simulink model "l512_devel_pps_2016f"  (R2012b)
settings: Solver=ode45  StartTime=0.0  StopTime=15000  RelTol=1e-3
undefined symbols (not defined in the file): sfp
libraries: xbsIndex_r4 x7383, casper_library_misc x259, casper_library_delays x118, xps_library x12, simulink x1
(part 14 of 82)

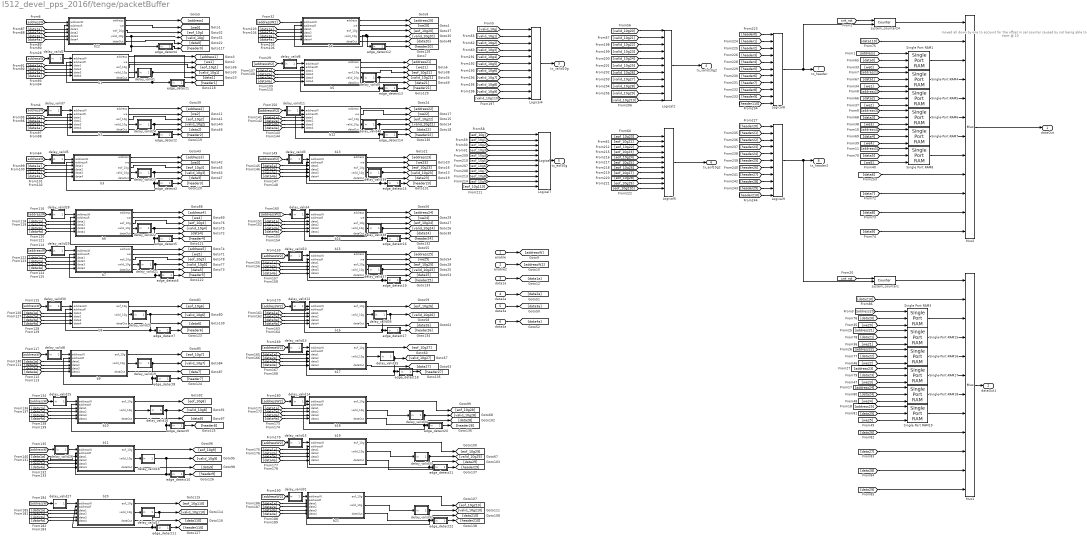
== system l512_devel_pps_2016f/tenge/packetBuffer ==
  note: moved all
      | down by one to account
      | for the offset in sel counter
      | caused by not being able to start @ 10
  enable : Inport
  enable2 : Inport  Port=2
  data1a : Inport  Port=3
  data2a : Inport  Port=4
  data3a : Inport  Port=5
  data4a : Inport  Port=6
  Logical{2,4,6..7} (4 alike) : xbsIndex_r4/Logical  logical_function=OR  inputs=11  en=off  latency=10  precision=Full  arith_type=Unsigned  n_bits=16  bin_pt=0  align_bp=on  dbl_ovrd=off  block_type=logical
      settings: block_version=11.4
  Logical8 : xbsIndex_r4/Logical  logical_function=OR  inputs=11  en=off  latency=5  precision=Full  arith_type=Unsigned  n_bits=16  bin_pt=0  align_bp=on  dbl_ovrd=off  block_type=logical
      settings: block_version=11.4
  Logical9 : xbsIndex_r4/Logical  logical_function=OR  inputs=11  en=off  latency=5  precision=Full  arith_type=Unsigned  n_bits=16  bin_pt=0  align_bp=on  dbl_ovrd=off  block_type=logical
      settings: block_version=11.4
  Mux1 : xbsIndex_r4/Mux  inputs=11  en=off  latency=2  precision=Full  arith_type="Signed  (2's comp)"  n_bits=8  bin_pt=2  quantization=Truncate  overflow=Wrap  dbl_ovrd=off  block_type=mux
      settings: xl_area=[0, 0, 0, 0, 0, 0, 0]
  Mux2 : xbsIndex_r4/Mux  inputs=11  en=off  latency=2  precision=Full  arith_type="Signed  (2's comp)"  n_bits=8  bin_pt=2  quantization=Truncate  overflow=Wrap  dbl_ovrd=off  block_type=mux
      settings: xl_area=[0, 0, 0, 0, 0, 0, 0]
  Single Port RAM{1,3..8,15..19} (12 alike) : xbsIndex_r4/Single Port RAM  depth=872  initVector=0  distributed_mem=Block RAM  write_mode=No Read On Write  rst=off  init_reg=0  en=off  latency=4  dbl_ovrd=off  optimize=Area  block_type=spram
  b1 : Subsystem
  b10 : Subsystem
  b11 : Subsystem
  b12 : Subsystem
  b13 : Subsystem
  b14 : Subsystem
  b15 : Subsystem
  b16 : Subsystem
  b17 : Subsystem
  b18 : Subsystem
  b19 : Subsystem
  b2 : Subsystem
  b20 : Subsystem
  b21 : Subsystem
  b22 : Subsystem
  b3 : Subsystem
  b4 : Subsystem
  b5 : Subsystem
  b6 : Subsystem
  b7 : Subsystem
  b8 : Subsystem
  b9 : Subsystem
  delay_valid1 : Subsystem  mask{delay=1166}
      mask prompts: delay "desired delay (>2)"
      mask Display: fprintf('Z^-%d', delay)
  delay_valid10 : Subsystem  mask{delay=1090}
      mask prompts: delay "desired delay (>2)"
      mask Display: fprintf('Z^-%d', delay)
  delay_valid11 : Subsystem  mask{delay=436}
      mask prompts: delay "desired delay (>2)"
      mask Display: fprintf('Z^-%d', delay)
  delay_valid12 : Subsystem  mask{delay=1308}
      mask prompts: delay "desired delay (>2)"
      mask Display: fprintf('Z^-%d', delay)
  delay_valid13 : Subsystem  mask{delay=1526}
      mask prompts: delay "desired delay (>2)"
      mask Display: fprintf('Z^-%d', delay)
  delay_valid14 : Subsystem  mask{delay=1744}
      mask prompts: delay "desired delay (>2)"
      mask Display: fprintf('Z^-%d', delay)
  delay_valid15 : Subsystem  mask{delay=1962}
      mask prompts: delay "desired delay (>2)"
      mask Display: fprintf('Z^-%d', delay)
  delay_valid16 : Subsystem  mask{delay=9328}
      mask prompts: delay "desired delay (>2)"
      mask Display: fprintf('Z^-%d', delay)
  delay_valid17 : Subsystem  mask{delay=11660}
      mask prompts: delay "desired delay (>2)"
      mask Display: fprintf('Z^-%d', delay)
  delay_valid18 : Subsystem  mask{delay=10494}
      mask prompts: delay "desired delay (>2)"
      mask Display: fprintf('Z^-%d', delay)
  delay_valid19 : Subsystem  mask{delay=8162}
      mask prompts: delay "desired delay (>2)"
      mask Display: fprintf('Z^-%d', delay)
  delay_valid2 : Subsystem  mask{delay=218}
      mask prompts: delay "desired delay (>2)"
      mask Display: fprintf('Z^-%d', delay)
  delay_valid20 : Subsystem  mask{delay=6996}
      mask prompts: delay "desired delay (>2)"
      mask Display: fprintf('Z^-%d', delay)
  delay_valid21 : Subsystem  mask{delay=5830}
      mask prompts: delay "desired delay (>2)"
      mask Display: fprintf('Z^-%d', delay)
  delay_valid22 : Subsystem  mask{delay=4664}
      mask prompts: delay "desired delay (>2)"
      mask Display: fprintf('Z^-%d', delay)
  delay_valid23 : Subsystem  mask{delay=3498}
      mask prompts: delay "desired delay (>2)"
      mask Display: fprintf('Z^-%d', delay)
  delay_valid24 : Subsystem  mask{delay=2332}
      mask prompts: delay "desired delay (>2)"
      mask Display: fprintf('Z^-%d', delay)
  delay_valid25 : Subsystem  mask{delay=1744}
      mask prompts: delay "desired delay (>2)"
      mask Display: fprintf('Z^-%d', delay)
  delay_valid26 : Subsystem  mask{delay=1962}
      mask prompts: delay "desired delay (>2)"
      mask Display: fprintf('Z^-%d', delay)
  delay_valid27 : Subsystem  mask{delay=2180}
      mask prompts: delay "desired delay (>2)"
      mask Display: fprintf('Z^-%d', delay)
  delay_valid28 : Subsystem  mask{delay=872}
      mask prompts: delay "desired delay (>2)"
      mask Display: fprintf('Z^-%d', delay)
  delay_valid29 : Subsystem  mask{delay=1090}
      mask prompts: delay "desired delay (>2)"
      mask Display: fprintf('Z^-%d', delay)
  delay_valid3 : Subsystem  mask{delay=654}
      mask prompts: delay "desired delay (>2)"
      mask Display: fprintf('Z^-%d', delay)
  delay_valid30 : Subsystem  mask{delay=1308}
      mask prompts: delay "desired delay (>2)"
      mask Display: fprintf('Z^-%d', delay)
  delay_valid31 : Subsystem  mask{delay=2180}
      mask prompts: delay "desired delay (>2)"
      mask Display: fprintf('Z^-%d', delay)
  delay_valid32 : Subsystem  mask{delay=11660}
      mask prompts: delay "desired delay (>2)"
      mask Display: fprintf('Z^-%d', delay)
  delay_valid33 : Subsystem  mask{delay=10494}
      mask prompts: delay "desired delay (>2)"
      mask Display: fprintf('Z^-%d', delay)
  delay_valid34 : Subsystem  mask{delay=9328}
      mask prompts: delay "desired delay (>2)"
      mask Display: fprintf('Z^-%d', delay)
  delay_valid35 : Subsystem  mask{delay=8162}
      mask prompts: delay "desired delay (>2)"
      mask Display: fprintf('Z^-%d', delay)
  delay_valid36 : Subsystem  mask{delay=6996}
      mask prompts: delay "desired delay (>2)"
      mask Display: fprintf('Z^-%d', delay)
  delay_valid37 : Subsystem  mask{delay=5830}
      mask prompts: delay "desired delay (>2)"
      mask Display: fprintf('Z^-%d', delay)
  delay_valid38 : Subsystem  mask{delay=4664}
      mask prompts: delay "desired delay (>2)"
      mask Display: fprintf('Z^-%d', delay)
  delay_valid39 : Subsystem  mask{delay=3498}
      mask prompts: delay "desired delay (>2)"
      mask Display: fprintf('Z^-%d', delay)
  delay_valid4 : Subsystem  mask{delay=872}
      mask prompts: delay "desired delay (>2)"
      mask Display: fprintf('Z^-%d', delay)
  delay_valid40 : Subsystem  mask{delay=2332}
      mask prompts: delay "desired delay (>2)"
      mask Display: fprintf('Z^-%d', delay)
  delay_valid5 : Subsystem  mask{delay=654}
      mask prompts: delay "desired delay (>2)"
      mask Display: fprintf('Z^-%d', delay)
  delay_valid6 : Subsystem  mask{delay=218}
      mask prompts: delay "desired delay (>2)"
      mask Display: fprintf('Z^-%d', delay)
  delay_valid7 : Subsystem  mask{delay=436}
      mask prompts: delay "desired delay (>2)"
      mask Display: fprintf('Z^-%d', delay)
  delay_valid8 : Subsystem  mask{delay=1526}
      mask prompts: delay "desired delay (>2)"
      mask Display: fprintf('Z^-%d', delay)
  delay_valid9 : Subsystem  mask{delay=1166}
      mask prompts: delay "desired delay (>2)"
      mask Display: fprintf('Z^-%d', delay)
  edge_detect1 : Subsystem  AncestorBlock=casper_library_misc/edge_detect  mask(edge_detect){edge=Rising, polarity=Active High, x_in=[0 0.08 0.08 0.16 0.16 0.24 0.24 0.32 0.32 0.4], y_in=[-1 -1  1  1  1  1  1  1  1  1], x_out=[0.6 0.68 0.68 0.76 0.76 0.84 0.84 0.92 0.92 1], y_out=[-1 -1  1  1 -1 -1 -1 -1 -1 -1]}
      mask prompts: edge "Edge Type"; polarity "Output Polarity"; x_in "Input X Positions"; y_in "Input Y Positions"; x_out "Output X Positions"; y_out "Output Y Positions"
      mask help: Output is active for one-cycle after each edge of the specified type (i.e. rising, falling or both).
      mask init: same as l512_devel_pps_2016f/tenge/chSel/edge_detect2
      settings: AttributesFormatString=|
      | rising edges
      | active high
      mask Help: Output is active for one-cycle after each edge of the specified type (i.e. rising, falling, or both).  Latency is zero.
      mask TypeOptions edge: Rising | Falling | Both
      mask TypeOptions polarity: Active High | Active Low
      mask Display:
      | plot(x_in_num,0.5+y_in_num*0.2);
      | plot(x_out_num,0.5+y_out_num*0.2);
  edge_detect10 : Subsystem  AncestorBlock=casper_library_misc/edge_detect  mask(edge_detect){edge=Rising, polarity=Active High, x_in=[0 0.08 0.08 0.16 0.16 0.24 0.24 0.32 0.32 0.4], y_in=[-1 -1  1  1  1  1  1  1  1  1], x_out=[0.6 0.68 0.68 0.76 0.76 0.84 0.84 0.92 0.92 1], y_out=[-1 -1  1  1 -1 -1 -1 -1 -1 -1]}
      mask prompts: edge "Edge Type"; polarity "Output Polarity"; x_in "Input X Positions"; y_in "Input Y Positions"; x_out "Output X Positions"; y_out "Output Y Positions"
      mask help: Output is active for one-cycle after each edge of the specified type (i.e. rising, falling or both).
      mask init: same as l512_devel_pps_2016f/tenge/chSel/edge_detect2
      settings: AttributesFormatString=|
      | rising edges
      | active high
      mask Help: Output is active for one-cycle after each edge of the specified type (i.e. rising, falling, or both).  Latency is zero.
      mask TypeOptions edge: Rising | Falling | Both
      mask TypeOptions polarity: Active High | Active Low
      mask Display:
      | plot(x_in_num,0.5+y_in_num*0.2);
      | plot(x_out_num,0.5+y_out_num*0.2);
  edge_detect11 : Subsystem  AncestorBlock=casper_library_misc/edge_detect  mask(edge_detect){edge=Rising, polarity=Active High, x_in=[0 0.08 0.08 0.16 0.16 0.24 0.24 0.32 0.32 0.4], y_in=[-1 -1  1  1  1  1  1  1  1  1], x_out=[0.6 0.68 0.68 0.76 0.76 0.84 0.84 0.92 0.92 1], y_out=[-1 -1  1  1 -1 -1 -1 -1 -1 -1]}
      mask prompts: edge "Edge Type"; polarity "Output Polarity"; x_in "Input X Positions"; y_in "Input Y Positions"; x_out "Output X Positions"; y_out "Output Y Positions"
      mask help: Output is active for one-cycle after each edge of the specified type (i.e. rising, falling or both).
      mask init: same as l512_devel_pps_2016f/tenge/chSel/edge_detect2
      settings: AttributesFormatString=|
      | rising edges
      | active high
      mask Help: Output is active for one-cycle after each edge of the specified type (i.e. rising, falling, or both).  Latency is zero.
      mask TypeOptions edge: Rising | Falling | Both
      mask TypeOptions polarity: Active High | Active Low
      mask Display:
      | plot(x_in_num,0.5+y_in_num*0.2);
      | plot(x_out_num,0.5+y_out_num*0.2);
  edge_detect12 : Subsystem  AncestorBlock=casper_library_misc/edge_detect  mask(edge_detect){edge=Rising, polarity=Active High, x_in=[0 0.08 0.08 0.16 0.16 0.24 0.24 0.32 0.32 0.4], y_in=[-1 -1  1  1  1  1  1  1  1  1], x_out=[0.6 0.68 0.68 0.76 0.76 0.84 0.84 0.92 0.92 1], y_out=[-1 -1  1  1 -1 -1 -1 -1 -1 -1]}
      mask prompts: edge "Edge Type"; polarity "Output Polarity"; x_in "Input X Positions"; y_in "Input Y Positions"; x_out "Output X Positions"; y_out "Output Y Positions"
      mask help: Output is active for one-cycle after each edge of the specified type (i.e. rising, falling or both).
      mask init: same as l512_devel_pps_2016f/tenge/chSel/edge_detect2
      settings: AttributesFormatString=|
      | rising edges
      | active high
      mask Help: Output is active for one-cycle after each edge of the specified type (i.e. rising, falling, or both).  Latency is zero.
      mask TypeOptions edge: Rising | Falling | Both
      mask TypeOptions polarity: Active High | Active Low
      mask Display:
      | plot(x_in_num,0.5+y_in_num*0.2);
      | plot(x_out_num,0.5+y_out_num*0.2);
  edge_detect13 : Subsystem  AncestorBlock=casper_library_misc/edge_detect  mask(edge_detect){edge=Rising, polarity=Active High, x_in=[0 0.08 0.08 0.16 0.16 0.24 0.24 0.32 0.32 0.4], y_in=[-1 -1  1  1  1  1  1  1  1  1], x_out=[0.6 0.68 0.68 0.76 0.76 0.84 0.84 0.92 0.92 1], y_out=[-1 -1  1  1 -1 -1 -1 -1 -1 -1]}
      mask prompts: edge "Edge Type"; polarity "Output Polarity"; x_in "Input X Positions"; y_in "Input Y Positions"; x_out "Output X Positions"; y_out "Output Y Positions"
      mask help: Output is active for one-cycle after each edge of the specified type (i.e. rising, falling or both).
      mask init: same as l512_devel_pps_2016f/tenge/chSel/edge_detect2
      settings: AttributesFormatString=|
      | rising edges
      | active high
      mask Help: Output is active for one-cycle after each edge of the specified type (i.e. rising, falling, or both).  Latency is zero.
      mask TypeOptions edge: Rising | Falling | Both
      mask TypeOptions polarity: Active High | Active Low
      mask Display:
      | plot(x_in_num,0.5+y_in_num*0.2);
      | plot(x_out_num,0.5+y_out_num*0.2);
  edge_detect14 : Subsystem  AncestorBlock=casper_library_misc/edge_detect  mask(edge_detect){edge=Rising, polarity=Active High, x_in=[0 0.08 0.08 0.16 0.16 0.24 0.24 0.32 0.32 0.4], y_in=[-1 -1  1  1  1  1  1  1  1  1], x_out=[0.6 0.68 0.68 0.76 0.76 0.84 0.84 0.92 0.92 1], y_out=[-1 -1  1  1 -1 -1 -1 -1 -1 -1]}
      mask prompts: edge "Edge Type"; polarity "Output Polarity"; x_in "Input X Positions"; y_in "Input Y Positions"; x_out "Output X Positions"; y_out "Output Y Positions"
      mask help: Output is active for one-cycle after each edge of the specified type (i.e. rising, falling or both).
      mask init: same as l512_devel_pps_2016f/tenge/chSel/edge_detect2
      settings: AttributesFormatString=|
      | rising edges
      | active high
      mask Help: Output is active for one-cycle after each edge of the specified type (i.e. rising, falling, or both).  Latency is zero.
      mask TypeOptions edge: Rising | Falling | Both
      mask TypeOptions polarity: Active High | Active Low
      mask Display:
      | plot(x_in_num,0.5+y_in_num*0.2);
      | plot(x_out_num,0.5+y_out_num*0.2);
  edge_detect15 : Subsystem  AncestorBlock=casper_library_misc/edge_detect  mask(edge_detect){edge=Rising, polarity=Active High, x_in=[0 0.08 0.08 0.16 0.16 0.24 0.24 0.32 0.32 0.4], y_in=[-1 -1  1  1  1  1  1  1  1  1], x_out=[0.6 0.68 0.68 0.76 0.76 0.84 0.84 0.92 0.92 1], y_out=[-1 -1  1  1 -1 -1 -1 -1 -1 -1]}
      mask prompts: edge "Edge Type"; polarity "Output Polarity"; x_in "Input X Positions"; y_in "Input Y Positions"; x_out "Output X Positions"; y_out "Output Y Positions"
      mask help: Output is active for one-cycle after each edge of the specified type (i.e. rising, falling or both).
      mask init: same as l512_devel_pps_2016f/tenge/chSel/edge_detect2
      settings: AttributesFormatString=|
      | rising edges
      | active high
      mask Help: Output is active for one-cycle after each edge of the specified type (i.e. rising, falling, or both).  Latency is zero.
      mask TypeOptions edge: Rising | Falling | Both
      mask TypeOptions polarity: Active High | Active Low
      mask Display:
      | plot(x_in_num,0.5+y_in_num*0.2);
      | plot(x_out_num,0.5+y_out_num*0.2);
  edge_detect16 : Subsystem  AncestorBlock=casper_library_misc/edge_detect  mask(edge_detect){edge=Rising, polarity=Active High, x_in=[0 0.08 0.08 0.16 0.16 0.24 0.24 0.32 0.32 0.4], y_in=[-1 -1  1  1  1  1  1  1  1  1], x_out=[0.6 0.68 0.68 0.76 0.76 0.84 0.84 0.92 0.92 1], y_out=[-1 -1  1  1 -1 -1 -1 -1 -1 -1]}
      mask prompts: edge "Edge Type"; polarity "Output Polarity"; x_in "Input X Positions"; y_in "Input Y Positions"; x_out "Output X Positions"; y_out "Output Y Positions"
      mask help: Output is active for one-cycle after each edge of the specified type (i.e. rising, falling or both).
      mask init: same as l512_devel_pps_2016f/tenge/chSel/edge_detect2
      settings: AttributesFormatString=|
      | rising edges
      | active high
      mask Help: Output is active for one-cycle after each edge of the specified type (i.e. rising, falling, or both).  Latency is zero.
      mask TypeOptions edge: Rising | Falling | Both
      mask TypeOptions polarity: Active High | Active Low
      mask Display:
      | plot(x_in_num,0.5+y_in_num*0.2);
      | plot(x_out_num,0.5+y_out_num*0.2);
  edge_detect17 : Subsystem  AncestorBlock=casper_library_misc/edge_detect  mask(edge_detect){edge=Rising, polarity=Active High, x_in=[0 0.08 0.08 0.16 0.16 0.24 0.24 0.32 0.32 0.4], y_in=[-1 -1  1  1  1  1  1  1  1  1], x_out=[0.6 0.68 0.68 0.76 0.76 0.84 0.84 0.92 0.92 1], y_out=[-1 -1  1  1 -1 -1 -1 -1 -1 -1]}
      mask prompts: edge "Edge Type"; polarity "Output Polarity"; x_in "Input X Positions"; y_in "Input Y Positions"; x_out "Output X Positions"; y_out "Output Y Positions"
      mask help: Output is active for one-cycle after each edge of the specified type (i.e. rising, falling or both).
      mask init: same as l512_devel_pps_2016f/tenge/chSel/edge_detect2
      settings: AttributesFormatString=|
      | rising edges
      | active high
      mask Help: Output is active for one-cycle after each edge of the specified type (i.e. rising, falling, or both).  Latency is zero.
      mask TypeOptions edge: Rising | Falling | Both
      mask TypeOptions polarity: Active High | Active Low
      mask Display:
      | plot(x_in_num,0.5+y_in_num*0.2);
      | plot(x_out_num,0.5+y_out_num*0.2);
  edge_detect18 : Subsystem  AncestorBlock=casper_library_misc/edge_detect  mask(edge_detect){edge=Rising, polarity=Active High, x_in=[0 0.08 0.08 0.16 0.16 0.24 0.24 0.32 0.32 0.4], y_in=[-1 -1  1  1  1  1  1  1  1  1], x_out=[0.6 0.68 0.68 0.76 0.76 0.84 0.84 0.92 0.92 1], y_out=[-1 -1  1  1 -1 -1 -1 -1 -1 -1]}
      mask prompts: edge "Edge Type"; polarity "Output Polarity"; x_in "Input X Positions"; y_in "Input Y Positions"; x_out "Output X Positions"; y_out "Output Y Positions"
      mask help: Output is active for one-cycle after each edge of the specified type (i.e. rising, falling or both).
      mask init: same as l512_devel_pps_2016f/tenge/chSel/edge_detect2
      settings: AttributesFormatString=|
      | rising edges
      | active high
      mask Help: Output is active for one-cycle after each edge of the specified type (i.e. rising, falling, or both).  Latency is zero.
      mask TypeOptions edge: Rising | Falling | Both
      mask TypeOptions polarity: Active High | Active Low
      mask Display:
      | plot(x_in_num,0.5+y_in_num*0.2);
      | plot(x_out_num,0.5+y_out_num*0.2);
  edge_detect19 : Subsystem  AncestorBlock=casper_library_misc/edge_detect  mask(edge_detect){edge=Rising, polarity=Active High, x_in=[0 0.08 0.08 0.16 0.16 0.24 0.24 0.32 0.32 0.4], y_in=[-1 -1  1  1  1  1  1  1  1  1], x_out=[0.6 0.68 0.68 0.76 0.76 0.84 0.84 0.92 0.92 1], y_out=[-1 -1  1  1 -1 -1 -1 -1 -1 -1]}
      mask prompts: edge "Edge Type"; polarity "Output Polarity"; x_in "Input X Positions"; y_in "Input Y Positions"; x_out "Output X Positions"; y_out "Output Y Positions"
      mask help: Output is active for one-cycle after each edge of the specified type (i.e. rising, falling or both).
      mask init: same as l512_devel_pps_2016f/tenge/chSel/edge_detect2
      settings: AttributesFormatString=|
      | rising edges
      | active high
      mask Help: Output is active for one-cycle after each edge of the specified type (i.e. rising, falling, or both).  Latency is zero.
      mask TypeOptions edge: Rising | Falling | Both
      mask TypeOptions polarity: Active High | Active Low
      mask Display:
      | plot(x_in_num,0.5+y_in_num*0.2);
      | plot(x_out_num,0.5+y_out_num*0.2);
  edge_detect2 : Subsystem  AncestorBlock=casper_library_misc/edge_detect  mask(edge_detect){edge=Rising, polarity=Active High, x_in=[0 0.08 0.08 0.16 0.16 0.24 0.24 0.32 0.32 0.4], y_in=[-1 -1  1  1  1  1  1  1  1  1], x_out=[0.6 0.68 0.68 0.76 0.76 0.84 0.84 0.92 0.92 1], y_out=[-1 -1  1  1 -1 -1 -1 -1 -1 -1]}
      mask prompts: edge "Edge Type"; polarity "Output Polarity"; x_in "Input X Positions"; y_in "Input Y Positions"; x_out "Output X Positions"; y_out "Output Y Positions"
      mask help: Output is active for one-cycle after each edge of the specified type (i.e. rising, falling or both).
      mask init: same as l512_devel_pps_2016f/tenge/chSel/edge_detect2
      settings: AttributesFormatString=|
      | rising edges
      | active high
      mask Help: Output is active for one-cycle after each edge of the specified type (i.e. rising, falling, or both).  Latency is zero.
      mask TypeOptions edge: Rising | Falling | Both
      mask TypeOptions polarity: Active High | Active Low
      mask Display:
      | plot(x_in_num,0.5+y_in_num*0.2);
      | plot(x_out_num,0.5+y_out_num*0.2);
  edge_detect20 : Subsystem  AncestorBlock=casper_library_misc/edge_detect  mask(edge_detect){edge=Rising, polarity=Active High, x_in=[0 0.08 0.08 0.16 0.16 0.24 0.24 0.32 0.32 0.4], y_in=[-1 -1  1  1  1  1  1  1  1  1], x_out=[0.6 0.68 0.68 0.76 0.76 0.84 0.84 0.92 0.92 1], y_out=[-1 -1  1  1 -1 -1 -1 -1 -1 -1]}
      mask prompts: edge "Edge Type"; polarity "Output Polarity"; x_in "Input X Positions"; y_in "Input Y Positions"; x_out "Output X Positions"; y_out "Output Y Positions"
      mask help: Output is active for one-cycle after each edge of the specified type (i.e. rising, falling or both).
      mask init: same as l512_devel_pps_2016f/tenge/chSel/edge_detect2
      settings: AttributesFormatString=|
      | rising edges
      | active high
      mask Help: Output is active for one-cycle after each edge of the specified type (i.e. rising, falling, or both).  Latency is zero.
      mask TypeOptions edge: Rising | Falling | Both
      mask TypeOptions polarity: Active High | Active Low
      mask Display:
      | plot(x_in_num,0.5+y_in_num*0.2);
      | plot(x_out_num,0.5+y_out_num*0.2);
  edge_detect21 : Subsystem  AncestorBlock=casper_library_misc/edge_detect  mask(edge_detect){edge=Rising, polarity=Active High, x_in=[0 0.08 0.08 0.16 0.16 0.24 0.24 0.32 0.32 0.4], y_in=[-1 -1  1  1  1  1  1  1  1  1], x_out=[0.6 0.68 0.68 0.76 0.76 0.84 0.84 0.92 0.92 1], y_out=[-1 -1  1  1 -1 -1 -1 -1 -1 -1]}
      mask prompts: edge "Edge Type"; polarity "Output Polarity"; x_in "Input X Positions"; y_in "Input Y Positions"; x_out "Output X Positions"; y_out "Output Y Positions"
      mask help: Output is active for one-cycle after each edge of the specified type (i.e. rising, falling or both).
      mask init: same as l512_devel_pps_2016f/tenge/chSel/edge_detect2
      settings: AttributesFormatString=|
      | rising edges
      | active high
      mask Help: Output is active for one-cycle after each edge of the specified type (i.e. rising, falling, or both).  Latency is zero.
      mask TypeOptions edge: Rising | Falling | Both
      mask TypeOptions polarity: Active High | Active Low
      mask Display:
      | plot(x_in_num,0.5+y_in_num*0.2);
      | plot(x_out_num,0.5+y_out_num*0.2);
  edge_detect22 : Subsystem  AncestorBlock=casper_library_misc/edge_detect  mask(edge_detect){edge=Rising, polarity=Active High, x_in=[0 0.08 0.08 0.16 0.16 0.24 0.24 0.32 0.32 0.4], y_in=[-1 -1  1  1  1  1  1  1  1  1], x_out=[0.6 0.68 0.68 0.76 0.76 0.84 0.84 0.92 0.92 1], y_out=[-1 -1  1  1 -1 -1 -1 -1 -1 -1]}
      mask prompts: edge "Edge Type"; polarity "Output Polarity"; x_in "Input X Positions"; y_in "Input Y Positions"; x_out "Output X Positions"; y_out "Output Y Positions"
      mask help: Output is active for one-cycle after each edge of the specified type (i.e. rising, falling or both).
      mask init: same as l512_devel_pps_2016f/tenge/chSel/edge_detect2
      settings: AttributesFormatString=|
      | rising edges
      | active high
      mask Help: Output is active for one-cycle after each edge of the specified type (i.e. rising, falling, or both).  Latency is zero.
      mask TypeOptions edge: Rising | Falling | Both
      mask TypeOptions polarity: Active High | Active Low
      mask Display:
      | plot(x_in_num,0.5+y_in_num*0.2);
      | plot(x_out_num,0.5+y_out_num*0.2);
  edge_detect3 : Subsystem  AncestorBlock=casper_library_misc/edge_detect  mask(edge_detect){edge=Rising, polarity=Active High, x_in=[0 0.08 0.08 0.16 0.16 0.24 0.24 0.32 0.32 0.4], y_in=[-1 -1  1  1  1  1  1  1  1  1], x_out=[0.6 0.68 0.68 0.76 0.76 0.84 0.84 0.92 0.92 1], y_out=[-1 -1  1  1 -1 -1 -1 -1 -1 -1]}
      mask prompts: edge "Edge Type"; polarity "Output Polarity"; x_in "Input X Positions"; y_in "Input Y Positions"; x_out "Output X Positions"; y_out "Output Y Positions"
      mask help: Output is active for one-cycle after each edge of the specified type (i.e. rising, falling or both).
      mask init: same as l512_devel_pps_2016f/tenge/chSel/edge_detect2
      settings: AttributesFormatString=|
      | rising edges
      | active high
      mask Help: Output is active for one-cycle after each edge of the specified type (i.e. rising, falling, or both).  Latency is zero.
      mask TypeOptions edge: Rising | Falling | Both
      mask TypeOptions polarity: Active High | Active Low
      mask Display:
      | plot(x_in_num,0.5+y_in_num*0.2);
      | plot(x_out_num,0.5+y_out_num*0.2);
  edge_detect4 : Subsystem  AncestorBlock=casper_library_misc/edge_detect  mask(edge_detect){edge=Rising, polarity=Active High, x_in=[0 0.08 0.08 0.16 0.16 0.24 0.24 0.32 0.32 0.4], y_in=[-1 -1  1  1  1  1  1  1  1  1], x_out=[0.6 0.68 0.68 0.76 0.76 0.84 0.84 0.92 0.92 1], y_out=[-1 -1  1  1 -1 -1 -1 -1 -1 -1]}
      mask prompts: edge "Edge Type"; polarity "Output Polarity"; x_in "Input X Positions"; y_in "Input Y Positions"; x_out "Output X Positions"; y_out "Output Y Positions"
      mask help: Output is active for one-cycle after each edge of the specified type (i.e. rising, falling or both).
      mask init: same as l512_devel_pps_2016f/tenge/chSel/edge_detect2
      settings: AttributesFormatString=|
      | rising edges
      | active high
      mask Help: Output is active for one-cycle after each edge of the specified type (i.e. rising, falling, or both).  Latency is zero.
      mask TypeOptions edge: Rising | Falling | Both
      mask TypeOptions polarity: Active High | Active Low
      mask Display:
      | plot(x_in_num,0.5+y_in_num*0.2);
      | plot(x_out_num,0.5+y_out_num*0.2);
  edge_detect5 : Subsystem  AncestorBlock=casper_library_misc/edge_detect  mask(edge_detect){edge=Rising, polarity=Active High, x_in=[0 0.08 0.08 0.16 0.16 0.24 0.24 0.32 0.32 0.4], y_in=[-1 -1  1  1  1  1  1  1  1  1], x_out=[0.6 0.68 0.68 0.76 0.76 0.84 0.84 0.92 0.92 1], y_out=[-1 -1  1  1 -1 -1 -1 -1 -1 -1]}
      mask prompts: edge "Edge Type"; polarity "Output Polarity"; x_in "Input X Positions"; y_in "Input Y Positions"; x_out "Output X Positions"; y_out "Output Y Positions"
      mask help: Output is active for one-cycle after each edge of the specified type (i.e. rising, falling or both).
      mask init: same as l512_devel_pps_2016f/tenge/chSel/edge_detect2
      settings: AttributesFormatString=|
      | rising edges
      | active high
      mask Help: Output is active for one-cycle after each edge of the specified type (i.e. rising, falling, or both).  Latency is zero.
      mask TypeOptions edge: Rising | Falling | Both
      mask TypeOptions polarity: Active High | Active Low
      mask Display:
      | plot(x_in_num,0.5+y_in_num*0.2);
      | plot(x_out_num,0.5+y_out_num*0.2);
  edge_detect6 : Subsystem  AncestorBlock=casper_library_misc/edge_detect  mask(edge_detect){edge=Rising, polarity=Active High, x_in=[0 0.08 0.08 0.16 0.16 0.24 0.24 0.32 0.32 0.4], y_in=[-1 -1  1  1  1  1  1  1  1  1], x_out=[0.6 0.68 0.68 0.76 0.76 0.84 0.84 0.92 0.92 1], y_out=[-1 -1  1  1 -1 -1 -1 -1 -1 -1]}
      mask prompts: edge "Edge Type"; polarity "Output Polarity"; x_in "Input X Positions"; y_in "Input Y Positions"; x_out "Output X Positions"; y_out "Output Y Positions"
      mask help: Output is active for one-cycle after each edge of the specified type (i.e. rising, falling or both).
      mask init: same as l512_devel_pps_2016f/tenge/chSel/edge_detect2
      settings: AttributesFormatString=|
      | rising edges
      | active high
      mask Help: Output is active for one-cycle after each edge of the specified type (i.e. rising, falling, or both).  Latency is zero.
      mask TypeOptions edge: Rising | Falling | Both
      mask TypeOptions polarity: Active High | Active Low
      mask Display:
      | plot(x_in_num,0.5+y_in_num*0.2);
      | plot(x_out_num,0.5+y_out_num*0.2);
  edge_detect7 : Subsystem  AncestorBlock=casper_library_misc/edge_detect  mask(edge_detect){edge=Rising, polarity=Active High, x_in=[0 0.08 0.08 0.16 0.16 0.24 0.24 0.32 0.32 0.4], y_in=[-1 -1  1  1  1  1  1  1  1  1], x_out=[0.6 0.68 0.68 0.76 0.76 0.84 0.84 0.92 0.92 1], y_out=[-1 -1  1  1 -1 -1 -1 -1 -1 -1]}
      mask prompts: edge "Edge Type"; polarity "Output Polarity"; x_in "Input X Positions"; y_in "Input Y Positions"; x_out "Output X Positions"; y_out "Output Y Positions"
      mask help: Output is active for one-cycle after each edge of the specified type (i.e. rising, falling or both).
      mask init: same as l512_devel_pps_2016f/tenge/chSel/edge_detect2
      settings: AttributesFormatString=|
      | rising edges
      | active high
      mask Help: Output is active for one-cycle after each edge of the specified type (i.e. rising, falling, or both).  Latency is zero.
      mask TypeOptions edge: Rising | Falling | Both
      mask TypeOptions polarity: Active High | Active Low
      mask Display:
      | plot(x_in_num,0.5+y_in_num*0.2);
      | plot(x_out_num,0.5+y_out_num*0.2);
  edge_detect8 : Subsystem  AncestorBlock=casper_library_misc/edge_detect  mask(edge_detect){edge=Rising, polarity=Active High, x_in=[0 0.08 0.08 0.16 0.16 0.24 0.24 0.32 0.32 0.4], y_in=[-1 -1  1  1  1  1  1  1  1  1], x_out=[0.6 0.68 0.68 0.76 0.76 0.84 0.84 0.92 0.92 1], y_out=[-1 -1  1  1 -1 -1 -1 -1 -1 -1]}
      mask prompts: edge "Edge Type"; polarity "Output Polarity"; x_in "Input X Positions"; y_in "Input Y Positions"; x_out "Output X Positions"; y_out "Output Y Positions"
      mask help: Output is active for one-cycle after each edge of the specified type (i.e. rising, falling or both).
      mask init: same as l512_devel_pps_2016f/tenge/chSel/edge_detect2
      settings: AttributesFormatString=|
      | rising edges
      | active high
      mask Help: Output is active for one-cycle after each edge of the specified type (i.e. rising, falling, or both).  Latency is zero.
      mask TypeOptions edge: Rising | Falling | Both
      mask TypeOptions polarity: Active High | Active Low
      mask Display:
      | plot(x_in_num,0.5+y_in_num*0.2);
      | plot(x_out_num,0.5+y_out_num*0.2);
  edge_detect9 : Subsystem  AncestorBlock=casper_library_misc/edge_detect  mask(edge_detect){edge=Rising, polarity=Active High, x_in=[0 0.08 0.08 0.16 0.16 0.24 0.24 0.32 0.32 0.4], y_in=[-1 -1  1  1  1  1  1  1  1  1], x_out=[0.6 0.68 0.68 0.76 0.76 0.84 0.84 0.92 0.92 1], y_out=[-1 -1  1  1 -1 -1 -1 -1 -1 -1]}
      mask prompts: edge "Edge Type"; polarity "Output Polarity"; x_in "Input X Positions"; y_in "Input Y Positions"; x_out "Output X Positions"; y_out "Output Y Positions"
      mask help: Output is active for one-cycle after each edge of the specified type (i.e. rising, falling or both).
      mask init: same as l512_devel_pps_2016f/tenge/chSel/edge_detect2
      settings: AttributesFormatString=|
      | rising edges
      | active high
      mask Help: Output is active for one-cycle after each edge of the specified type (i.e. rising, falling, or both).  Latency is zero.
      mask TypeOptions edge: Rising | Falling | Both
      mask TypeOptions polarity: Active High | Active Low
      mask Display:
      | plot(x_in_num,0.5+y_in_num*0.2);
      | plot(x_out_num,0.5+y_out_num*0.2);
  system_counter1 : xbsIndex_r4/Counter  cnt_type=Count Limited  cnt_to=10  operation=Up  start_count=0  cnt_by_val=1  arith_type=Unsigned  n_bits=4  bin_pt=0  load_pin=off  rst=on  en=on  explicit_period=on  period=1  dbl_ovrd=off  use_behavioral_HDL=off  implementation=Fabric  block_type=counter
      settings: block_version=11.4
  system_counter24 : xbsIndex_r4/Counter  cnt_type=Count Limited  cnt_to=10  operation=Up  start_count=0  cnt_by_val=1  arith_type=Unsigned  n_bits=4  bin_pt=0  load_pin=off  rst=on  en=on  explicit_period=on  period=1  dbl_ovrd=off  use_behavioral_HDL=off  implementation=Fabric  block_type=counter
      settings: block_version=11.4
  dataOut : Outport
  dataOut1 : Outport  Port=2
  tx_valid10g : Outport  Port=3
  tx_valid10g2 : Outport  Port=4
  tx_eof10g : Outport  Port=5
  tx_eof10g2 : Outport  Port=6
  tx_header : Outport  Port=7
  tx_header2 : Outport  Port=8
  wires:
  [data110] -> Mux2/2
  Single Port RAM1/1 -> Mux2/3
  Single Port RAM4/1 -> Mux2/4
  Single Port RAM5/1 -> Mux2/5
  Single Port RAM6/1 -> Mux2/6
  Single Port RAM7/1 -> Mux2/7
  Single Port RAM8/1 -> Mux2/8
  [data7] -> Mux2/10
  [data8] -> Mux2/11
  [data9] -> Mux2/12
  Mux2/1 -> dataOut/1
  [data210] -> Mux1/2
  Single Port RAM3/1 -> Mux1/3
  Single Port RAM15/1 -> Mux1/4
  Single Port RAM16/1 -> Mux1/5
  Single Port RAM17/1 -> Mux1/6
  Single Port RAM18/1 -> Mux1/7
  Single Port RAM19/1 -> Mux1/8
  [data26] -> Mux1/9
  [data27] -> Mux1/10
  [data28] -> Mux1/11
  [data29] -> Mux1/12
  Mux1/1 -> dataOut1/1
  enable/1 -> [addressW]
  enable2/1 -> [addressW2]
  [addressW] -> b22/1(addressW)
  b22/1(address) -> [address]
  b22/2(we) -> [we0]
  [addressW] -> delay_valid2/1(in)
  b1/1(address) -> [address1]
  b1/2(we) -> [we1]
  b4/1(address) -> [address20]
  [addressW2] -> delay_valid6/1(in)
  [valid_10g] -> Logical4/1
  [valid_10g1] -> Logical4/2
  Logical4/1 -> tx_valid10g/1
  [valid_10g20] -> Logical2/1
  [valid_10g21] -> Logical2/2
  Logical2/1 -> tx_valid10g2/1
  [eof_10g] -> Logical7/1
  [eof_10g1] -> Logical7/2
  Logical7/1 -> tx_eof10g/1
  [eof_10g20] -> Logical6/1
  [eof_10g21] -> Logical6/2
  Logical6/1 -> tx_eof10g2/1
  b4/2(we) -> [we20]
  b1/4(valid_10g) -> delay_valid1/1(in)
  b4/4(valid_10g) -> [valid_10g20], b4/2(addressR), edge_detect12/1(in)
  b4/3(eof_10g) -> [eof_10g20]
  [addressW] -> delay_valid7/1(in)
  b2/1(address) -> [address2]
  b2/2(we) -> [we2]
  b2/4(valid_10g) -> delay_valid24/1(in)
  b2/3(eof_10g) -> [eof_10g2]
  [eof_10g2] -> Logical7/3
  [eof_10g3] -> Logical7/4
  [valid_10g2] -> Logical4/3
  [valid_10g3] -> Logical4/4
  [addressW] -> delay_valid5/1(in)
  delay_valid6/1(out) -> b5/1(addressW)
  delay_valid2/1(out) -> b1/1(addressW)
  [addressW2] -> b4/1(addressW)
  b22/5(dataOut) -> [data0]
  b1/5(dataOut) -> [data1]
  b2/5(dataOut) -> [data2]
  b4/5(dataOut) -> [data20]
  data1a/1 -> [data1a]
  data2a/1 -> [data2a]
  data3a/1 -> [data3a]
  data4a/1 -> [data4a]
  [data1a] -> b22/3(data1)
  [data2a] -> b22/4(data2)
  [data3a] -> b22/5(data3)
  [data4a] -> b22/6(data4)
  [data1a] -> b1/3(data1)
  [data2a] -> b1/4(data2)
  [data3a] -> b1/5(data3)
  [data4a] -> b1/6(data4)
  [data1a] -> b2/3(data1)
  [data2a] -> b2/4(data2)
  [data3a] -> b2/5(data3)
  [data4a] -> b2/6(data4)
  [data1a] -> b3/3(data1)
  [data2a] -> b3/4(data2)
  [data3a] -> b3/5(data3)
  [data4a] -> b3/6(data4)
  [data1a] -> b4/3(data1)
  [data2a] -> b4/4(data2)
  [data3a] -> b4/5(data3)
  [data4a] -> b4/6(data4)
  [data1a] -> b5/3(data1)
  [data2a] -> b5/4(data2)
  [data3a] -> b5/5(data3)
  [data4a] -> b5/6(data4)
  [addressW] -> delay_valid28/1(in)
  [addressW] -> delay_valid29/1(in)
  [addressW] -> delay_valid30/1(in)
  b8/2(valid_10g) -> delay_valid20/1(in)
  b8/1(eof_10g) -> [eof_10g6]
  [addressW] -> delay_valid8/1(in)
  delay_valid29/1(out) -> b7/1(addressW)
  b8/3(dataOut) -> [data6]
  [data1a] -> b6/3(data1)
  [data2a] -> b6/4(data2)
  [data3a] -> b6/5(data3)
  [data4a] -> b6/6(data4)
  [data1a] -> b7/3(data1)
  [data2a] -> b7/4(data2)
  [data3a] -> b7/5(data3)
  [data4a] -> b7/6(data4)
  [data1a] -> b8/3(data1)
  [data2a] -> b8/4(data2)
  [data3a] -> b8/5(data3)
  [data4a] -> b8/6(data4)
  [data1a] -> b9/3(data1)
  [data2a] -> b9/4(data2)
  [data3a] -> b9/5(data3)
  [data4a] -> b9/6(data4)
  [addressW] -> delay_valid25/1(in)
  [addressW] -> delay_valid26/1(in)
  [data1a] -> b10/3(data1)
  [data2a] -> b10/4(data2)
  [data3a] -> b10/5(data3)
  [data4a] -> b10/6(data4)
  [data1a] -> b11/3(data1)
  [data2a] -> b11/4(data2)
  [data3a] -> b11/5(data3)
  [data4a] -> b11/6(data4)
  [addressW2] -> delay_valid3/1(in)
  delay_valid3/1(out) -> b13/1(addressW)
  [addressW2] -> delay_valid11/1(in)
  [data1a] -> b12/3(data1)
  [data2a] -> b12/4(data2)
  [data3a] -> b12/5(data3)
  [data4a] -> b12/6(data4)
  [data1a] -> b13/3(data1)
  [data2a] -> b13/4(data2)
  [data3a] -> b13/5(data3)
  [data4a] -> b13/6(data4)
  [addressW2] -> delay_valid10/1(in)
  delay_valid10/1(out) -> b15/1(addressW)
  [addressW2] -> delay_valid4/1(in)
  [data1a] -> b14/3(data1)
  [data2a] -> b14/4(data2)
  [data3a] -> b14/5(data3)
  [data4a] -> b14/6(data4)
  [data1a] -> b15/3(data1)
  [data2a] -> b15/4(data2)
  [data3a] -> b15/5(data3)
  [data4a] -> b15/6(data4)
  [addressW2] -> delay_valid13/1(in)
  delay_valid13/1(out) -> b17/1(addressW)
  [addressW2] -> delay_valid12/1(in)
  [data1a] -> b16/3(data1)
  [data2a] -> b16/4(data2)
  [data3a] -> b16/5(data3)
  [data4a] -> b16/6(data4)
  [data1a] -> b17/3(data1)
  [data2a] -> b17/4(data2)
  [data3a] -> b17/5(data3)
  [data4a] -> b17/6(data4)
  [addressW2] -> delay_valid15/1(in)
  delay_valid15/1(out) -> b19/1(addressW)
  [addressW2] -> delay_valid14/1(in)
  [data1a] -> b18/3(data1)
  [data2a] -> b18/4(data2)
  [data3a] -> b18/5(data3)
  [data4a] -> b18/6(data4)
  [data1a] -> b19/3(data1)
  [data2a] -> b19/4(data2)
  [data3a] -> b19/5(data3)
  [data4a] -> b19/6(data4)
  [addressW] -> delay_valid27/1(in)
  [data1a] -> b20/3(data1)
  [data2a] -> b20/4(data2)
  [data3a] -> b20/5(data3)
  [data4a] -> b20/6(data4)
  [addressW2] -> delay_valid31/1(in)
  delay_valid31/1(out) -> b21/1(addressW)
  [data1a] -> b21/3(data1)
  [data2a] -> b21/4(data2)
  [data3a] -> b21/5(data3)
  [data4a] -> b21/6(data4)
  [valid_10g4] -> Logical4/5
  [valid_10g5] -> Logical4/6
  [valid_10g6] -> Logical4/7
  [valid_10g7] -> Logical4/8
  [valid_10g8] -> Logical4/9
  [valid_10g9] -> Logical4/10
  [valid_10g110] -> Logical4/11
  [valid_10g22] -> Logical2/3
  [valid_10g23] -> Logical2/4
  [valid_10g24] -> Logical2/5
  [valid_10g25] -> Logical2/6
  [valid_10g26] -> Logical2/7
  [valid_10g27] -> Logical2/8
  [valid_10g28] -> Logical2/9
  [valid_10g29] -> Logical2/10
  [valid_10g210] -> Logical2/11
  [eof_10g4] -> Logical7/5
  [eof_10g5] -> Logical7/6
  [eof_10g6] -> Logical7/7
  [eof_10g7] -> Logical7/8
  [eof_10g8] -> Logical7/9
  [eof_10g9] -> Logical7/10
  [eof_10g110] -> Logical7/11
  [eof_10g22] -> Logical6/3
  [eof_10g23] -> Logical6/4
  [eof_10g24] -> Logical6/5
  [eof_10g25] -> Logical6/6
  [eof_10g26] -> Logical6/7
  [eof_10g27] -> Logical6/8
  [eof_10g28] -> Logical6/9
  [eof_10g29] -> Logical6/10
  [eof_10g210] -> Logical6/11
  [header0] -> Logical8/1
  [header1] -> Logical8/2
  [header2] -> Logical8/3
  [header3] -> Logical8/4
  [header4] -> Logical8/5
  [header5] -> Logical8/6
  [header6] -> Logical8/7
  [header7] -> Logical8/8
  [header8] -> Logical8/9
  [header9] -> Logical8/10
  [header110] -> Logical8/11
  Logical8/1 -> tx_header/1, system_counter24/2
  [header20] -> Logical9/1
  [header21] -> Logical9/2
  [header22] -> Logical9/3
  [header23] -> Logical9/4
  [header24] -> Logical9/5
  [header25] -> Logical9/6
  [header26] -> Logical9/7
  [header27] -> Logical9/8
  [header28] -> Logical9/9
  [header29] -> Logical9/10
  [header210] -> Logical9/11
  Logical9/1 -> tx_header2/1, system_counter1/2
  edge_detect4/1(out) -> [header0]
  delay_valid7/1(out) -> b2/1(addressW)
  delay_valid5/1(out) -> b3/1(addressW)
  delay_valid28/1(out) -> b6/1(addressW)
  delay_valid30/1(out) -> b8/1(addressW)
  delay_valid8/1(out) -> b9/1(addressW)
  delay_valid25/1(out) -> b10/1(addressW)
  delay_valid26/1(out) -> b11/1(addressW)
  delay_valid27/1(out) -> b20/1(addressW)
  delay_valid11/1(out) -> b12/1(addressW)
  delay_valid4/1(out) -> b14/1(addressW)
  delay_valid12/1(out) -> b16/1(addressW)
  delay_valid14/1(out) -> b18/1(addressW)
  edge_detect1/1(out) -> [header1]
  edge_detect7/1(out) -> [header6]
  edge_detect12/1(out) -> [header20]
  system_counter24/1 -> Mux2/1
  system_counter1/1 -> Mux1/1
  [cnt_rst] -> system_counter24/1
  [cnt_rst] -> system_counter1/1
  delay_valid24/1(out) -> [valid_10g2], b2/2(addressR), edge_detect2/1(in)
  edge_detect2/1(out) -> [header2]
  b3/1(address) -> [address3]
  b3/2(we) -> [we3]
  b3/5(dataOut) -> [data3]
  delay_valid23/1(out) -> [valid_10g3], b3/2(addressR), edge_detect3/1(in)
  b3/3(eof_10g) -> [eof_10g3]
  b3/4(valid_10g) -> delay_valid23/1(in)
  edge_detect3/1(out) -> [header3]
  b6/5(dataOut) -> [data4]
  delay_valid22/1(out) -> b6/2(addressR), edge_detect5/1(in), [valid_10g4]
  b6/3(eof_10g) -> [eof_10g4]
  b6/4(valid_10g) -> delay_valid22/1(in)
  edge_detect5/1(out) -> [header4]
  b6/1(address) -> [address4]
  b6/2(we) -> [we4]
  b7/1(address) -> [address5]
  b7/2(we) -> [we5]
  b7/5(dataOut) -> [data5]
  delay_valid21/1(out) -> [valid_10g5], b7/2(addressR), edge_detect6/1(in)
  b7/3(eof_10g) -> [eof_10g5]
  b7/4(valid_10g) -> delay_valid21/1(in)
  edge_detect6/1(out) -> [header5]
  b9/3(dataOut) -> [data7]
  delay_valid19/1(out) -> b9/2(addressR), edge_detect8/1(in), [valid_10g7]
  b9/2(valid_10g) -> delay_valid19/1(in)
  edge_detect8/1(out) -> [header7]
  b10/3(dataOut) -> [data8]
  delay_valid16/1(out) -> b10/2(addressR), edge_detect9/1(in), [valid_10g8]
  b10/1(eof_10g) -> [eof_10g8]
  b10/2(valid_10g) -> delay_valid16/1(in)
  edge_detect9/1(out) -> [header8]
  b11/3(dataOut) -> [data9]
  delay_valid18/1(out) -> [valid_10g9], b11/2(addressR), edge_detect10/1(in)
  b11/2(valid_10g) -> delay_valid18/1(in)
  edge_detect10/1(out) -> [header9]
  b20/3(dataOut) -> [data110]
  delay_valid17/1(out) -> b20/2(addressR), edge_detect11/1(in), [valid_10g110]
  b20/2(valid_10g) -> delay_valid17/1(in)
  edge_detect11/1(out) -> [header110]
  b5/1(address) -> [address21]
  b5/2(we) -> [we21]
  b5/5(dataOut) -> [data21]
  delay_valid9/1(out) -> b5/2(addressR), edge_detect13/1(in), [valid_10g21]
  b5/3(eof_10g) -> [eof_10g21]
  b5/4(valid_10g) -> delay_valid9/1(in)
  edge_detect13/1(out) -> [header21]
  b12/1(address) -> [address22]
  b12/2(we) -> [we22]
  b12/5(dataOut) -> [data22]
  delay_valid40/1(out) -> b12/2(addressR), edge_detect14/1(in), [valid_10g22]
  edge_detect14/1(out) -> [header22]
  b12/3(eof_10g) -> [eof_10g22]
  b12/4(valid_10g) -> delay_valid40/1(in)
  b13/1(address) -> [address23]
  b13/2(we) -> [we23]
  b13/5(dataOut) -> [data23]
  delay_valid39/1(out) -> b13/2(addressR), edge_detect15/1(in), [valid_10g23]
  edge_detect15/1(out) -> [header23]
  b13/3(eof_10g) -> [eof_10g23]
  b13/4(valid_10g) -> delay_valid39/1(in)
  b14/1(address) -> [address24]
  b14/2(we) -> [we24]
  b14/5(dataOut) -> [data24]
  delay_valid38/1(out) -> b14/2(addressR), edge_detect16/1(in), [valid_10g24]
  edge_detect16/1(out) -> [header24]
  b16/3(dataOut) -> [data26]
  delay_valid36/1(out) -> b16/2(addressR), edge_detect17/1(in), [valid_10g26]
  edge_detect17/1(out) -> [header26]
  b17/3(dataOut) -> [data27]
  delay_valid35/1(out) -> b17/2(addressR), edge_detect18/1(in), [valid_10g27]
  edge_detect18/1(out) -> [header27]
  b15/1(address) -> [address25]
  b15/2(we) -> [we25]
  b15/5(dataOut) -> [data25]
  delay_valid37/1(out) -> b15/2(addressR), edge_detect19/1(in), [valid_10g25]
  edge_detect19/1(out) -> [header25]
  b14/3(eof_10g) -> [eof_10g24]
  b14/4(valid_10g) -> delay_valid38/1(in)
  b15/4(valid_10g) -> delay_valid37/1(in)
  b15/3(eof_10g) -> [eof_10g25]
  b16/2(valid_10g) -> delay_valid36/1(in)
  b17/1(eof_10g) -> [eof_10g27]
  b17/2(valid_10g) -> delay_valid35/1(in)
  b18/3(dataOut) -> [data28]
  delay_valid34/1(out) -> [valid_10g28], b18/2(addressR), edge_detect20/1(in)
  edge_detect20/1(out) -> [header28]
  b19/3(dataOut) -> [data29]
  delay_valid33/1(out) -> b19/2(addressR), edge_detect21/1(in), [valid_10g29]
  edge_detect21/1(out) -> [header29]
  b21/3(dataOut) -> [data210]
  delay_valid32/1(out) -> b21/2(addressR), edge_detect22/1(in), [valid_10g210]
  edge_detect22/1(out) -> [header210]
  b21/2(valid_10g) -> delay_valid32/1(in)
  b19/2(valid_10g) -> delay_valid33/1(in)
  b18/2(valid_10g) -> delay_valid34/1(in)
  delay_valid20/1(out) -> b8/2(addressR), edge_detect7/1(in), [valid_10g6]
  [address] -> Single Port RAM1/1
  [address1] -> Single Port RAM4/1
  [address2] -> Single Port RAM5/1
  [address3] -> Single Port RAM6/1
  [address4] -> Single Port RAM7/1
  [address5] -> Single Port RAM8/1
  [we0] -> Single Port RAM1/3
  [we1] -> Single Port RAM4/3
  [we2] -> Single Port RAM5/3
  [we3] -> Single Port RAM6/3
  [we4] -> Single Port RAM7/3
  [we5] -> Single Port RAM8/3
  [data0] -> Single Port RAM1/2
  [data1] -> Single Port RAM4/2
  [data2] -> Single Port RAM5/2
  [data3] -> Single Port RAM6/2
  [data4] -> Single Port RAM7/2
  [data5] -> Single Port RAM8/2
  [address20] -> Single Port RAM3/1
  [address21] -> Single Port RAM15/1
  [address23] -> Single Port RAM17/1
  [address24] -> Single Port RAM18/1
  [address25] -> Single Port RAM19/1
  [address22] -> Single Port RAM16/1
  [we20] -> Single Port RAM3/3
  [we21] -> Single Port RAM15/3
  [we22] -> Single Port RAM16/3
  [we23] -> Single Port RAM17/3
  [we24] -> Single Port RAM18/3
  [we25] -> Single Port RAM19/3
  [data20] -> Single Port RAM3/2
  [data21] -> Single Port RAM15/2
  [data22] -> Single Port RAM16/2
  [data23] -> Single Port RAM17/2
  [data24] -> Single Port RAM18/2
  [data25] -> Single Port RAM19/2
  b1/3(eof_10g) -> [eof_10g1]
  delay_valid1/1(out) -> [valid_10g1], edge_detect1/1(in), b1/2(addressR)
  b22/4(valid_10g) -> b22/2(addressR), edge_detect4/1(in), [valid_10g]
  b22/3(eof_10g) -> [eof_10g]
  [data6] -> Mux2/9
  b9/1(eof_10g) -> [eof_10g7]
  b11/1(eof_10g) -> [eof_10g9]
  b20/1(eof_10g) -> [eof_10g110]
  b16/1(eof_10g) -> [eof_10g26]
  b18/1(eof_10g) -> [eof_10g28]
  b19/1(eof_10g) -> [eof_10g29]
  b21/1(eof_10g) -> [eof_10g210]

== system l512_devel_pps_2016f/tenge/pipeline1 ==
  d : Inport
  Register0 : xbsIndex_r4/Register  init=0  rst=off  en=off  dbl_ovrd=off  block_type=register
      settings: block_version=11.4
  q : Outport
  wires:
  d/1 -> Register0/1
  Register0/1 -> q/1

== system l512_devel_pps_2016f/tenge/pipeline10 ==
  d : Inport
  Register0 : xbsIndex_r4/Register  init=0  rst=off  en=off  dbl_ovrd=off  block_type=register
      settings: block_version=11.4
  q : Outport
  wires:
  Register0/1 -> q/1
  d/1 -> Register0/1

== system l512_devel_pps_2016f/tenge/pipeline11 ==
  d : Inport
  Register0 : xbsIndex_r4/Register  init=0  rst=off  en=off  dbl_ovrd=off  block_type=register
      settings: block_version=11.4
  q : Outport
  wires:
  d/1 -> Register0/1
  Register0/1 -> q/1

== system l512_devel_pps_2016f/tenge/pipeline12 ==
  d : Inport
  Register0 : xbsIndex_r4/Register  init=0  rst=off  en=off  dbl_ovrd=off  block_type=register
      settings: block_version=11.4
  q : Outport
  wires:
  Register0/1 -> q/1
  d/1 -> Register0/1

== system l512_devel_pps_2016f/tenge/pipeline13 ==
  d : Inport
  Register0 : xbsIndex_r4/Register  init=0  rst=off  en=off  dbl_ovrd=off  block_type=register
      settings: block_version=11.4
  q : Outport
  wires:
  d/1 -> Register0/1
  Register0/1 -> q/1

== system l512_devel_pps_2016f/tenge/pipeline14 ==
  d : Inport
  Register0 : xbsIndex_r4/Register  init=0  rst=off  en=off  dbl_ovrd=off  block_type=register
      settings: block_version=11.4
  q : Outport
  wires:
  Register0/1 -> q/1
  d/1 -> Register0/1

== system l512_devel_pps_2016f/tenge/pipeline15 ==
  d : Inport
  Register0 : xbsIndex_r4/Register  init=0  rst=off  en=off  dbl_ovrd=off  block_type=register
      settings: block_version=11.4
  q : Outport
  wires:
  Register0/1 -> q/1
  d/1 -> Register0/1

== system l512_devel_pps_2016f/tenge/pipeline16 ==
  d : Inport
  Register0 : xbsIndex_r4/Register  init=0  rst=off  en=off  dbl_ovrd=off  block_type=register
      settings: block_version=11.4
  q : Outport
  wires:
  d/1 -> Register0/1
  Register0/1 -> q/1

== system l512_devel_pps_2016f/tenge/pipeline17 ==
  d : Inport
  Register0 : xbsIndex_r4/Register  init=0  rst=off  en=off  dbl_ovrd=off  block_type=register
      settings: block_version=11.4
  q : Outport
  wires:
  Register0/1 -> q/1
  d/1 -> Register0/1

== system l512_devel_pps_2016f/tenge/pipeline18 ==
  d : Inport
  Register0 : xbsIndex_r4/Register  init=0  rst=off  en=off  dbl_ovrd=off  block_type=register
      settings: block_version=11.4
  q : Outport
  wires:
  d/1 -> Register0/1
  Register0/1 -> q/1

== system l512_devel_pps_2016f/tenge/pipeline19 ==
  d : Inport
  Register0 : xbsIndex_r4/Register  init=0  rst=off  en=off  dbl_ovrd=off  block_type=register
      settings: block_version=11.4
  q : Outport
  wires:
  Register0/1 -> q/1
  d/1 -> Register0/1

== system l512_devel_pps_2016f/tenge/pipeline2 ==
  d : Inport
  Register0 : xbsIndex_r4/Register  init=0  rst=off  en=off  dbl_ovrd=off  block_type=register
      settings: block_version=11.4
  q : Outport
  wires:
  Register0/1 -> q/1
  d/1 -> Register0/1
